simulink model "Klimaanlage"  (R2023b)
settings: Solver=FixedStepAuto  StartTime=0.0  StopTime=40000  RelTol=1e-3  EnableMultiTasking=on
undefined symbols (not defined in the file or in its folder): C, K_p, LowerUserTemp, R, T_a, T_i_start, T_n
libraries: mbedblockslib x11, simulink_extras x1
settings Model: ExtModeTrigDuration=10  Creator=kilia  LastModifiedBy=kilia
settings OptimizationCC: UseDivisionForNetSlopeComputation=on  GainParamInheritBuiltInType=on  UseFloatMulNetSlope=on  PassReuseOutputArgsAs=Individual arguments  ZeroExternalMemoryAtStartup=off  ZeroInternalMemoryAtStartup=off  NoFixptDivByZeroProtection=on  EfficientFloat2IntCast=on  LifeSpan=1  MaxStackSize=64  OptimizeBlockOrder=speed  DifferentSizesBufferReuse=on  EfficientTunableParamExpr=on
settings DebuggingCC: ParameterTunabilityLossMsg=error
settings HardwareCC: ProdBitPerPointer=32  ProdBitPerSizeT=32  ProdBitPerPtrDiffT=32  ProdLargestAtomicInteger=Long  ProdLargestAtomicFloat=Double  ProdWordSize=32  ProdLongLongMode=on  ProdHWDeviceType=ARM Compatible->ARM Cortex
settings SFSimCC: MATLABDynamicMemAlloc=off
settings RTWCC: Description=Embedded Coder  SystemTargetFile=ert.tlc  HardwareBoard=STM32 Nucleo F103RB  TemplateMakefile=ert_default_tmf  Toolchain=GNU Tools for ARM Embedded Processors
settings CodeAppCC: ForceParamTrailComments=on  IgnoreCustomStorageClasses=off  OperatorAnnotations=on  SimulinkDataObjDesc=on  SFDataObjDesc=on  CustomSymbolStrGlobalVar=rt$N$M  CustomSymbolStrType=$N$M  CustomSymbolStrFcn=$N$M$F  CustomSymbolStrMacro=$N$M  InsertBlockDesc=on
settings ERTTargetCC: IncludeMdlTerminateFcn=off  CombineSignalStateStructs=on  SupportComplex=off  SupportContinuousTime=on  ExtModeTransport=3  ExtModeStaticAlloc=on  ExtModeStaticAllocSize=2000  ExtModeMexFile=ext_xcp  ExtModeIntrfLevel=Level2 - Open  ERTFilePackagingFormat=CompactWithDataFile

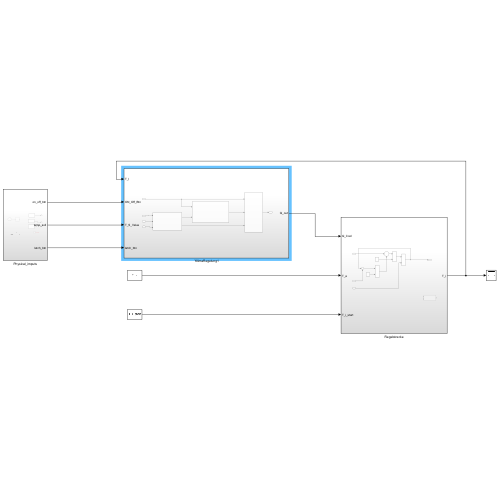
[thumbnail: Simulink's stored preview of the top-level diagram]
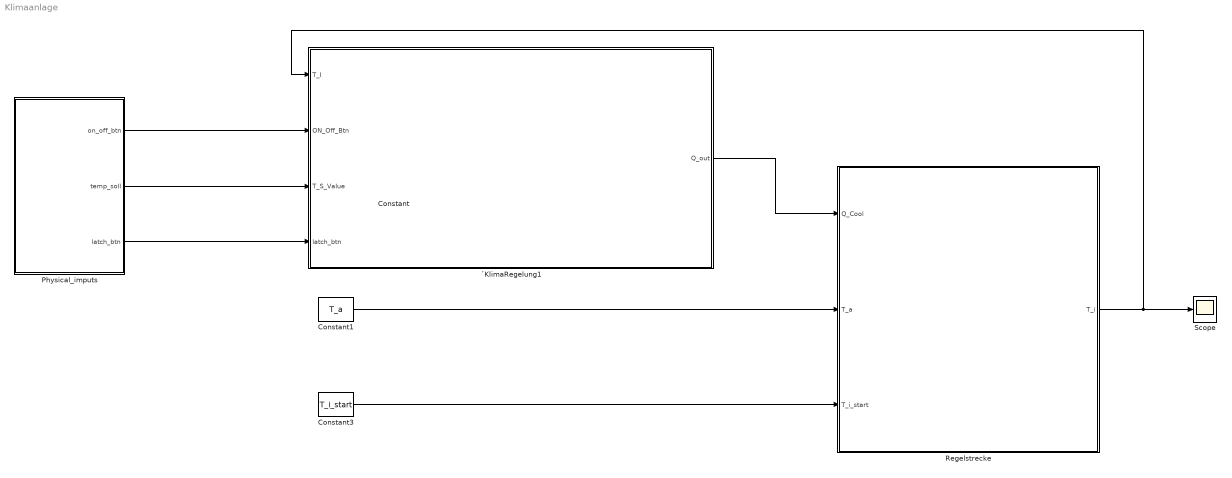
== system Klimaanlage ==
  Constant : Constant  Value=15
  Constant1 : Constant  Value=T_a
  Constant3 : Constant  Value=T_i_start
  Physical_imputs : Subsystem
  Regelstrecke : Subsystem
  Scope : Scope
  ´KlimaRegelung1 : Subsystem
  wires:
  Regelstrecke/1(T_i) -> ´KlimaRegelung1/1(T_I), Scope/1
  Constant1/1 -> Regelstrecke/2(T_a)
  ´KlimaRegelung1/1(Q_out) -> Regelstrecke/1(Q_Cool)
  Constant3/1 -> Regelstrecke/3(T_i_start)
  Physical_imputs/1(on_off_btn) -> ´KlimaRegelung1/2(ON_Off_Btn)
  Physical_imputs/3(latch_btn) -> ´KlimaRegelung1/4(latch_btn)
  Physical_imputs/2(temp_soll) -> ´KlimaRegelung1/3(T_S_Value)

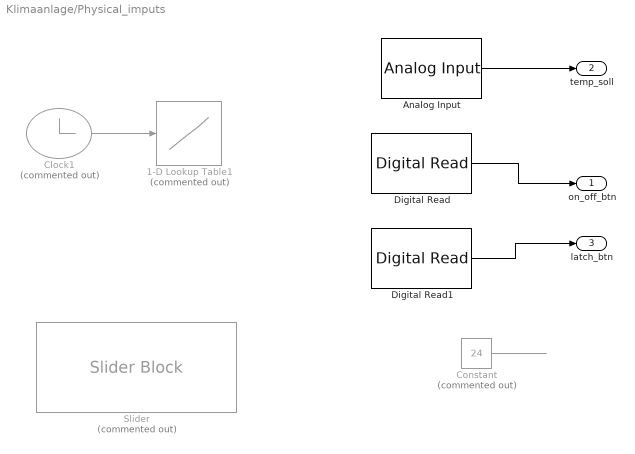
== system Klimaanlage/Physical_imputs ==
  1-D Lookup Table1 : Lookup_n-D  Commented=on  NumberOfTableDimensions=1  BreakpointsForDimension1=[1;50;51;300;301;400;401]  Table=[1;1;0;0;1;1;0]  InternalRulePriority=Speed  RndMeth=Simplest
  Analog Input : mbedblockslib/Analog Input  Pin=A0  ReadResultsOnly=off  ConversionTriggerSource=Software  ExternalTriggerType=uint32( 0 )  OutputDataType=double  EnableConversionCompleteNotify=off  EnableOuputStatus=off  SampleTime=-1
      settings: LibrarySourceBlock=stmnucleorootlib/Common/Analog Input
  Clock1 : Clock  Commented=on
  Constant : Constant  Commented=on  Value=24
  Digital Read : mbedblockslib/Digital Read  Pin=D2  Direction=input  SampleTime=-1
      settings: LibrarySourceBlock=stmnucleorootlib/Common/Digital Read
  Digital Read1 : mbedblockslib/Digital Read  Pin=D3  Direction=input  SampleTime=-1
      settings: LibrarySourceBlock=stmnucleorootlib/Common/Digital Read
  Slider : SliderBlock  Commented=on  ScaleMin=16  ScaleMax=28
  on_off_btn : Outport
  temp_soll : Outport  Port=2
  latch_btn : Outport  Port=3
  wires:
  Clock1/1 -> 1-D Lookup Table1/1
  Constant/1 -> ?
  Digital Read/1 -> on_off_btn/1
  Digital Read1/1 -> latch_btn/1
  Analog Input/1 -> temp_soll/1

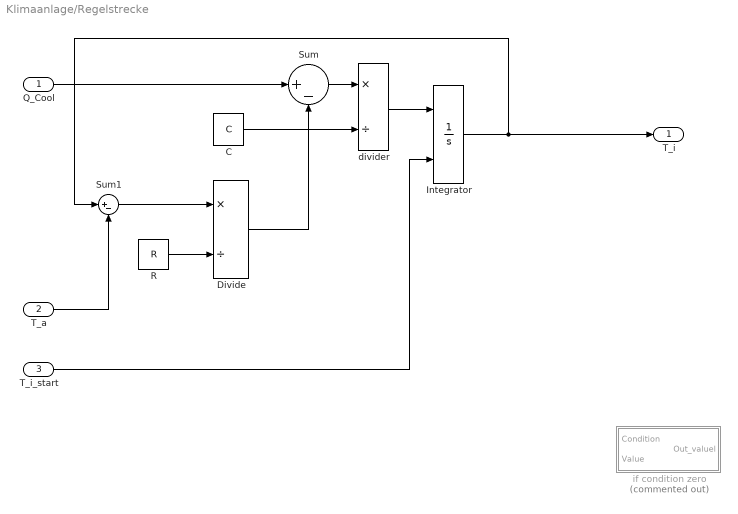
== system Klimaanlage/Regelstrecke ==
  Q_Cool : Inport
  T_a : Inport  Port=2
  T_i_start : Inport  Port=3
  C : Constant  Value=C
  Divide : Product  Inputs=*/
  Integrator : Integrator  InitialConditionSource=external
  R : Constant  Value=R
  Sum : Sum  Inputs=|+-
  Sum1 : Sum  Inputs=|+-
  divider : Product  Inputs=*/
  if condition zero : Subsystem  Commented=on
  T_i : Outport
  wires:
  Sum/1 -> divider/1
  Sum1/1 -> Divide/1
  divider/1 -> Integrator/1
  R/1 -> Divide/2
  C/1 -> divider/2
  Q_Cool/1 -> Sum/1
  Divide/1 -> Sum/2
  T_a/1 -> Sum1/2
  Integrator/1 -> Sum1/1, T_i/1
  T_i_start/1 -> Integrator/2

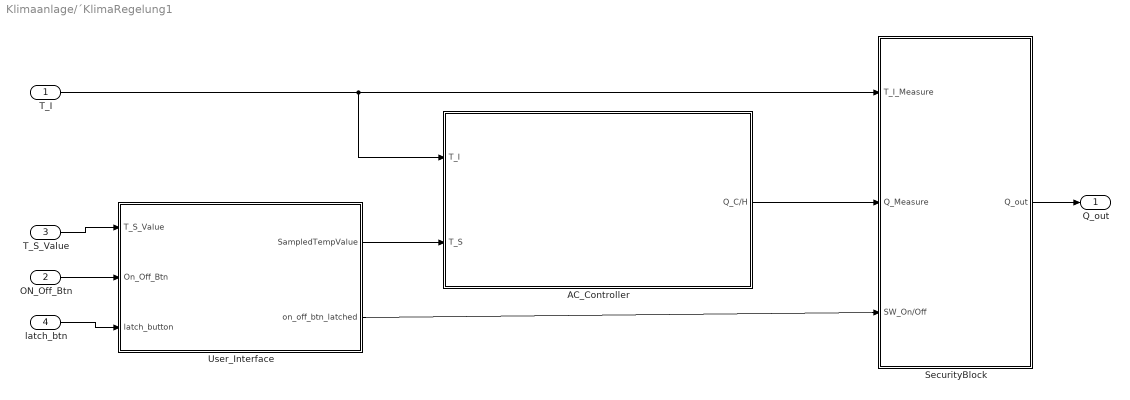
== system Klimaanlage/´KlimaRegelung1 ==
  T_I : Inport
  ON_Off_Btn : Inport  Port=2
  T_S_Value : Inport  Port=3
  latch_btn : Inport  Port=4
  AC_Controller : Subsystem
  SecurityBlock : Subsystem
  User_Interface : Subsystem
  Q_out : Outport
  wires:
  T_I/1 -> AC_Controller/1(T_I), SecurityBlock/1(T_I_Measure)
  User_Interface/2(on_off_btn_latched) -> SecurityBlock/3(SW_On/Off)
  User_Interface/1(SampledTempValue) -> AC_Controller/2(T_S)
  ON_Off_Btn/1 -> User_Interface/2(On_Off_Btn)
  T_S_Value/1 -> User_Interface/1(T_S_Value)
  AC_Controller/1(Q_C/H) -> SecurityBlock/2(Q_Measure)
  SecurityBlock/1(Q_out) -> Q_out/1
  latch_btn/1 -> User_Interface/3(latch_button)

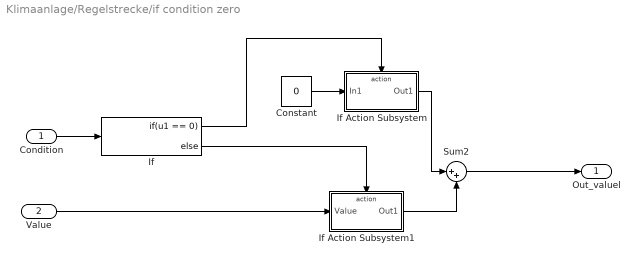
== system Klimaanlage/Regelstrecke/if condition zero ==
  Condition : Inport
  Value : Inport  Port=2
  Constant : Constant  Value=0
  If : If  IfExpression=u1 == 0
  If Action Subsystem : Subsystem  TreatAsAtomicUnit=on
  If Action Subsystem1 : Subsystem  TreatAsAtomicUnit=on
  Sum2 : Sum  Inputs=|++
  Out_valuel : Outport
  wires:
  Sum2/1 -> Out_valuel/1
  If/2 -> If Action Subsystem1/Action
  If Action Subsystem1/1(Out1) -> Sum2/2
  If/1 -> If Action Subsystem/Action
  If Action Subsystem/1(Out1) -> Sum2/1
  Condition/1 -> If/1
  Value/1 -> If Action Subsystem1/1(Value)
  Constant/1 -> If Action Subsystem/1(In1)

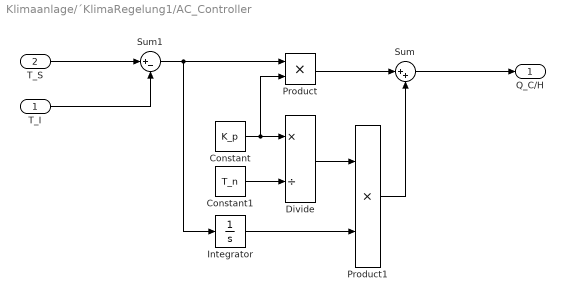
== system Klimaanlage/´KlimaRegelung1/AC_Controller ==
  T_I : Inport
  T_S : Inport  Port=2
  Constant : Constant  Value=K_p
  Constant1 : Constant  Value=T_n
  Divide : Product  Inputs=*/
  Integrator : Integrator
  Product : Product
  Product1 : Product
  Sum : Sum  Inputs=|++
  Sum1 : Sum  Inputs=|+-
  Q_C/H : Outport
  wires:
  Integrator/1 -> Product1/2
  Product/1 -> Sum/1
  Product1/1 -> Sum/2
  Sum1/1 -> Integrator/1, Product/1
  T_S/1 -> Sum1/1
  T_I/1 -> Sum1/2
  Constant/1 -> Product/2, Divide/1
  Constant1/1 -> Divide/2
  Divide/1 -> Product1/1
  Sum/1 -> Q_C/H/1

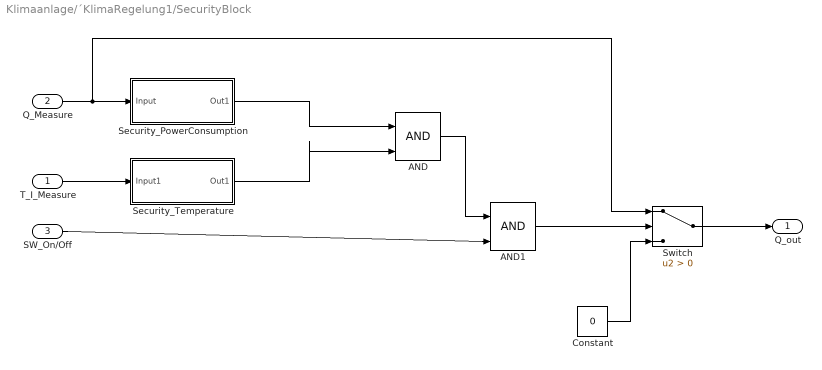
== system Klimaanlage/´KlimaRegelung1/SecurityBlock ==
  T_I_Measure : Inport
  Q_Measure : Inport  Port=2
  SW_On/Off : Inport  Port=3
  AND : Logic  IconShape=distinctive  AllPortsSameDT=off  OutDataTypeStr=boolean
  AND1 : Logic  IconShape=distinctive  AllPortsSameDT=off  OutDataTypeStr=boolean
  Constant : Constant  Value=0
  Security_PowerConsumption : Subsystem
  Security_Temperature : Subsystem
  Switch : Switch  Criteria=u2 > Threshold  SaturateOnIntegerOverflow=off  InputSameDT=off
  Q_out : Outport
  wires:
  Q_Measure/1 -> Switch/1, Security_PowerConsumption/1(Input)
  T_I_Measure/1 -> Security_Temperature/1(Input1)
  Security_PowerConsumption/1(Out1) -> AND/1
  Security_Temperature/1(Out1) -> AND/2
  AND1/1 -> Switch/2
  SW_On/Off/1 -> AND1/2
  Switch/1 -> Q_out/1
  Constant/1 -> Switch/3
  AND/1 -> AND1/1

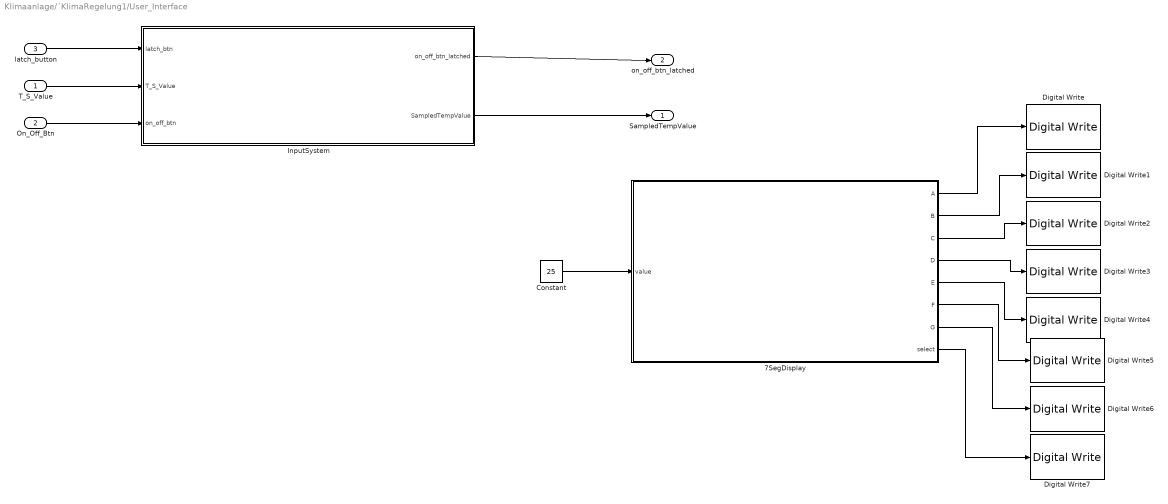
== system Klimaanlage/´KlimaRegelung1/User_Interface ==
  T_S_Value : Inport
  On_Off_Btn : Inport  Port=2
  latch_button : Inport  Port=3
  7SegDisplay : Subsystem
  Constant : Constant  Value=25
  Digital Write : mbedblockslib/Digital Write  Pin=PA_5  Direction=output
      settings: LibrarySourceBlock=stmnucleorootlib/Common/Digital Write
  Digital Write1 : mbedblockslib/Digital Write  Pin=PA_6  Direction=output
      settings: LibrarySourceBlock=stmnucleorootlib/Common/Digital Write
  Digital Write2 : mbedblockslib/Digital Write  Pin=PA_7  Direction=output
      settings: LibrarySourceBlock=stmnucleorootlib/Common/Digital Write
  Digital Write3 : mbedblockslib/Digital Write  Pin=PA_8  Direction=output
      settings: LibrarySourceBlock=stmnucleorootlib/Common/Digital Write
  Digital Write4 : mbedblockslib/Digital Write  Pin=PA_9  Direction=output
      settings: LibrarySourceBlock=stmnucleorootlib/Common/Digital Write
  Digital Write5 : mbedblockslib/Digital Write  Pin=PA_15  Direction=output
      settings: LibrarySourceBlock=stmnucleorootlib/Common/Digital Write
  Digital Write6 : mbedblockslib/Digital Write  Pin=PB_9  Direction=output
      settings: LibrarySourceBlock=stmnucleorootlib/Common/Digital Write
  Digital Write7 : mbedblockslib/Digital Write  Pin=PB_0  Direction=output
      settings: LibrarySourceBlock=stmnucleorootlib/Common/Digital Write
  InputSystem : Subsystem
  SampledTempValue : Outport
  on_off_btn_latched : Outport  Port=2
  wires:
  InputSystem/1(on_off_btn_latched) -> on_off_btn_latched/1
  T_S_Value/1 -> InputSystem/2(T_S_Value)
  On_Off_Btn/1 -> InputSystem/3(on_off_btn)
  7SegDisplay/1(A) -> Digital Write/1
  7SegDisplay/2(B) -> Digital Write1/1
  7SegDisplay/3(C) -> Digital Write2/1
  7SegDisplay/4(D) -> Digital Write3/1
  7SegDisplay/5(E) -> Digital Write4/1
  7SegDisplay/6(F) -> Digital Write5/1
  7SegDisplay/7(G) -> Digital Write6/1
  7SegDisplay/8(select) -> Digital Write7/1
  latch_button/1 -> InputSystem/1(latch_btn)
  InputSystem/2(SampledTempValue) -> SampledTempValue/1
  Constant/1 -> 7SegDisplay/1(value)

== system Klimaanlage/Regelstrecke/if condition zero/If Action Subsystem ==
  In1 : Inport
  Action Port : ActionPort  ActionPortLabel=if(u1 == 0)
  Out1 : Outport
  wires:
  In1/1 -> Out1/1

== system Klimaanlage/Regelstrecke/if condition zero/If Action Subsystem1 ==
  Value : Inport
  Action Port : ActionPort  ActionPortLabel=else
  Out1 : Outport
  wires:
  Value/1 -> Out1/1

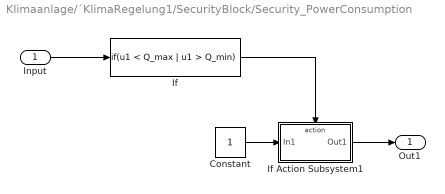
== system Klimaanlage/´KlimaRegelung1/SecurityBlock/Security_PowerConsumption ==
  Input : Inport
  Constant : Constant
  If : If  IfExpression=u1 < Q_max | u1 > Q_min  ShowElse=off
  If Action Subsystem1 : Subsystem  TreatAsAtomicUnit=on
  Out1 : Outport
  wires:
  Input/1 -> If/1
  If/1 -> If Action Subsystem1/Action
  If Action Subsystem1/1(Out1) -> Out1/1
  Constant/1 -> If Action Subsystem1/1(In1)

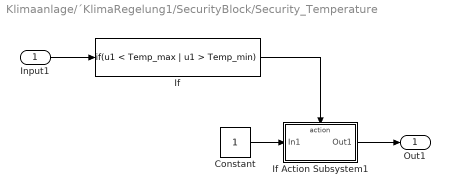
== system Klimaanlage/´KlimaRegelung1/SecurityBlock/Security_Temperature ==
  Input1 : Inport
  Constant : Constant
  If : If  IfExpression=u1 < Temp_max | u1 > Temp_min  ShowElse=off
  If Action Subsystem1 : Subsystem  TreatAsAtomicUnit=on
  Out1 : Outport
  wires:
  Input1/1 -> If/1
  Constant/1 -> If Action Subsystem1/1(In1)
  If Action Subsystem1/1(Out1) -> Out1/1
  If/1 -> If Action Subsystem1/Action

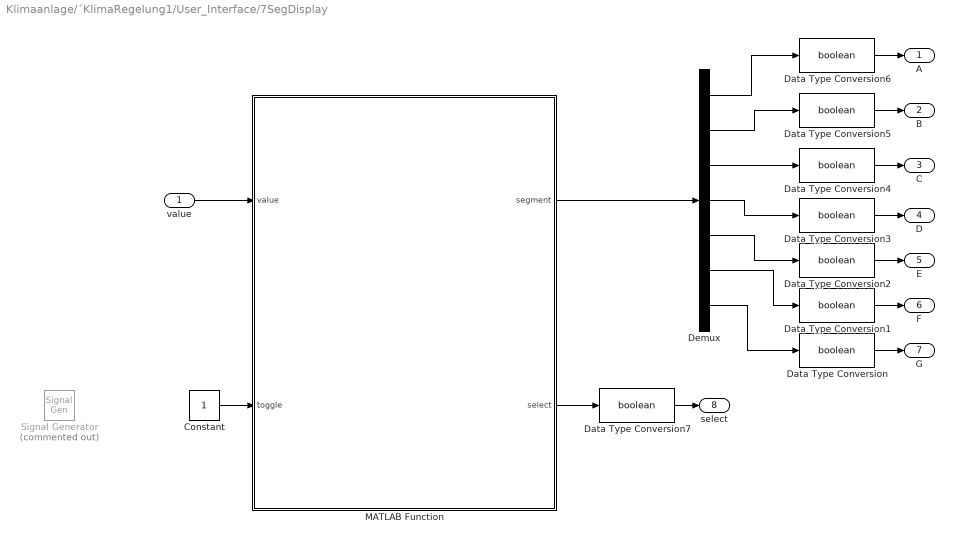
== system Klimaanlage/´KlimaRegelung1/User_Interface/7SegDisplay ==
  value : Inport
  Constant : Constant
  Data Type Conversion{,1..7} (8 alike) : DataTypeConversion  OutDataTypeStr=boolean  SaturateOnIntegerOverflow=off  RndMeth=Floor
  Demux : Demux  Outputs=7
  MATLAB Function : MATLAB Function  TreatAsAtomicUnit=on
  Signal Generator : SignalGenerator  Commented=on  WaveForm=square  Frequency=100
  A : Outport
  B : Outport  Port=2
  C : Outport  Port=3
  D : Outport  Port=4
  E : Outport  Port=5
  F : Outport  Port=6
  G : Outport  Port=7
  select : Outport  Port=8
  wires:
  MATLAB Function/1(segment) -> Demux/1
  MATLAB Function/2(select) -> Data Type Conversion7/1
  value/1 -> MATLAB Function/1(value)
  Demux/1 -> Data Type Conversion6/1
  Demux/2 -> Data Type Conversion5/1
  Demux/3 -> Data Type Conversion4/1
  Demux/4 -> Data Type Conversion3/1
  Demux/5 -> Data Type Conversion2/1
  Demux/6 -> Data Type Conversion1/1
  Demux/7 -> Data Type Conversion/1
  Data Type Conversion/1 -> G/1
  Data Type Conversion6/1 -> A/1
  Data Type Conversion5/1 -> B/1
  Data Type Conversion4/1 -> C/1
  Data Type Conversion3/1 -> D/1
  Data Type Conversion2/1 -> E/1
  Data Type Conversion1/1 -> F/1
  Data Type Conversion7/1 -> select/1
  Constant/1 -> MATLAB Function/2(toggle)

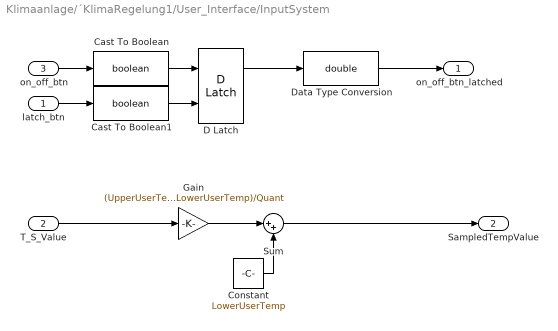
== system Klimaanlage/´KlimaRegelung1/User_Interface/InputSystem ==
  latch_btn : Inport
  T_S_Value : Inport  Port=2
  on_off_btn : Inport  Port=3
  Cast To Boolean : DataTypeConversion  OutDataTypeStr=boolean  SaturateOnIntegerOverflow=off  RndMeth=Floor
  Cast To Boolean1 : DataTypeConversion  OutDataTypeStr=boolean  SaturateOnIntegerOverflow=off  RndMeth=Floor
  Constant : Constant  Value=LowerUserTemp
  D Latch : simulink_extras/Flip Flops/D Latch
  Data Type Conversion : DataTypeConversion  OutDataTypeStr=double  SaturateOnIntegerOverflow=off  RndMeth=Floor
  Gain : Gain  Gain=(UpperUserTemp - LowerUserTemp)/Quant  OutDataTypeStr=int32
  Sum : Sum  Inputs=|++
  on_off_btn_latched : Outport
  SampledTempValue : Outport  Port=2
  wires:
  D Latch/1 -> Data Type Conversion/1
  latch_btn/1 -> Cast To Boolean1/1
  T_S_Value/1 -> Gain/1
  Cast To Boolean/1 -> D Latch/1
  Cast To Boolean1/1 -> D Latch/2
  Data Type Conversion/1 -> on_off_btn_latched/1
  on_off_btn/1 -> Cast To Boolean/1
  Gain/1 -> Sum/1
  Sum/1 -> SampledTempValue/1
  Constant/1 -> Sum/2

== system Klimaanlage/´KlimaRegelung1/SecurityBlock/Security_PowerConsumption/If Action Subsystem1 ==
  In1 : Inport
  Action Port : ActionPort  ActionPortLabel=if(u1 < Q_max | u1 > Q_min)
  Out1 : Outport
  wires:
  In1/1 -> Out1/1

== system Klimaanlage/´KlimaRegelung1/SecurityBlock/Security_Temperature/If Action Subsystem1 ==
  In1 : Inport
  Action Port : ActionPort  ActionPortLabel=if(u1 < Temp_max | u1 > Temp_min)
  Out1 : Outport
  wires:
  In1/1 -> Out1/1

== matlab function Klimaanlage/´KlimaRegelung1/User_Interface/7SegDisplay/MATLAB Function ==
  data: segment output; value input; toggle input; select output
function [segment, select] = SevenSegmentControl(value, toggle)
% Eingänge:
% value: Zahlenwert (0–99), der angezeigt werden soll
% toggle: Umschaltsignal (0 oder 1) zum Wechsel zwischen Zehner- und Einerstelle

% Ausgänge:
% segment: 8-Bit-Signal für die Segmente (a-g und dp)
% select: 2-Bit-Signal zur Aktivierung eines Displays

% Begrenzung des Werts auf den Bereich 0–99
value = max(0, min(99, value));

% Segment-Codes für 0–9 (a-g, dp: [abcdefg.dp])
segments = [
    0,1,1,1,1,1,1; % 0
    0,0,0,0,1,1,0; % 1
    1,0,1,1,0,1,1; % 2
    0,0,0,1,1,1,1; % 3
    1,1,0,0,1,1,0; % 4
    1,1,0,1,1,0,1; % 5
    1,1,1,1,1,0,1; % 6
    0,0,0,0,1,1,1; % 7
    1,1,1,1,1,1,1; % 8
    1,1,0,1,1,1,1; % 9
];

% Zerlege den Wert in Zehner- und Einerstelle
tens = floor(value / 10);
ones = mod(value, 10);

% Anzeigelogik basierend auf toggle
if toggle == 1
    segment = segments(tens + 1,:); % Zehnerstelle
    select = 0; % Aktiviert das erste Display
else
    segment = segments(ones + 1,:); % Einerstelle
    select = 1; % Aktiviert das zweite Display
end
end
